simulink model "modelo_SI"  (R2019b)
settings: Solver=VariableStepAuto  StartTime=0.0  StopTime=365  RelTol=1e-3
settings Model: Creator=lucia  LastModifiedBy=lucia

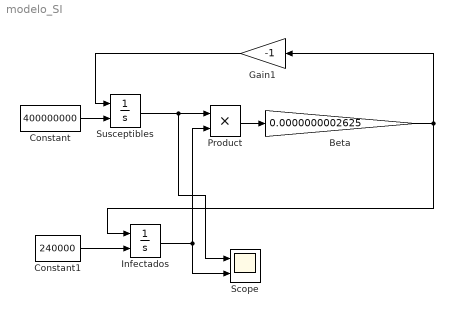
== system modelo_SI ==
  Beta : Gain  Gain=0.0000000002625
  Constant : Constant  Value=400000000
  Constant1 : Constant  Value=240000
  Gain1 : Gain  Gain=-1
  Infectados : Integrator  InitialConditionSource=external  InitialCondition=10
  Product : Product
  Scope : Scope  NumInputPorts=2
  Susceptibles : Integrator  InitialConditionSource=external  InitialCondition=990
  wires:
  Infectados/1 -> Scope/2, Product/2
  Susceptibles/1 -> Scope/1, Product/1
  Product/1 -> Beta/1
  Beta/1 -> Gain1/1, Infectados/1
  Gain1/1 -> Susceptibles/1
  Constant/1 -> Susceptibles/2
  Constant1/1 -> Infectados/2
